simulink model "BiNode2016a"  (R2016a)
settings: Solver=ode4  StartTime=0.0  StopTime=6  FixedStep=tstep  RelTol=1e-3
PreLoadFcn:
  | xred=rednoise(20*1000)
model workspace (MAT data in the model file):
  P1 = Simulink.Parameter
  P1.Value = 4.5
  P1.DataType = 'auto'
  P1.Dimensions = [1 1]
  P2 = Simulink.Parameter
  P2.Value = 0
  P2.DataType = 'auto'
  P2.Dimensions = [1 1]
  V = Simulink.Parameter
  V.Value = 0.5
  V.DataType = 'auto'
  V.Dimensions = [1 1]
  e0 = Simulink.Parameter
  e0.Value = 2.5
  e0.DataType = 'auto'
  e0.Dimensions = [1 1]
  kp = Simulink.Parameter
  kp.Value = 0.1
  kp.DataType = 'auto'
  kp.Dimensions = [1 1]
  r = Simulink.Parameter
  r.Value = 1.12
  r.DataType = 'auto'
  r.Dimensions = [1 1]
  tao = Simulink.Parameter
  tao.Value = 0.01
  tao.DataType = 'auto'
  tao.Dimensions = [1 1]
  tstep = Simulink.Parameter
  tstep.Value = 0.0001
  tstep.DataType = 'auto'
  tstep.Dimensions = [1 1]
  v0 = Simulink.Parameter
  v0.Value = 5
  v0.DataType = 'auto'
  v0.Dimensions = [1 1]
libraries: commnoisgen2 x2
settings Model: Creator=u0085294  LastModifiedBy=mchehelc
settings DataIOCC: LimitDataPoints=on  SaveFormat=Array
settings OptimizationCC: ExpressionDepthLimit=2147483647
settings DebuggingCC: UnderspecifiedInitializationDetection=Classic  MergeDetectMultiDrivingBlocksExec=none  SolverPrmCheckMsg=warning  StateNameClashWarn=warning
settings HardwareCC: ProdBitPerPointer=32  ProdLargestAtomicFloat=None  ProdIntDivRoundTo=Undefined  ProdEndianess=Unspecified  ProdWordSize=32  ProdHWDeviceType=32-bit Generic
settings ModelReferenceCC: PropagateSignalLabelsOutOfModel=off
settings ConfigComp: CovModelRefEnable=Off

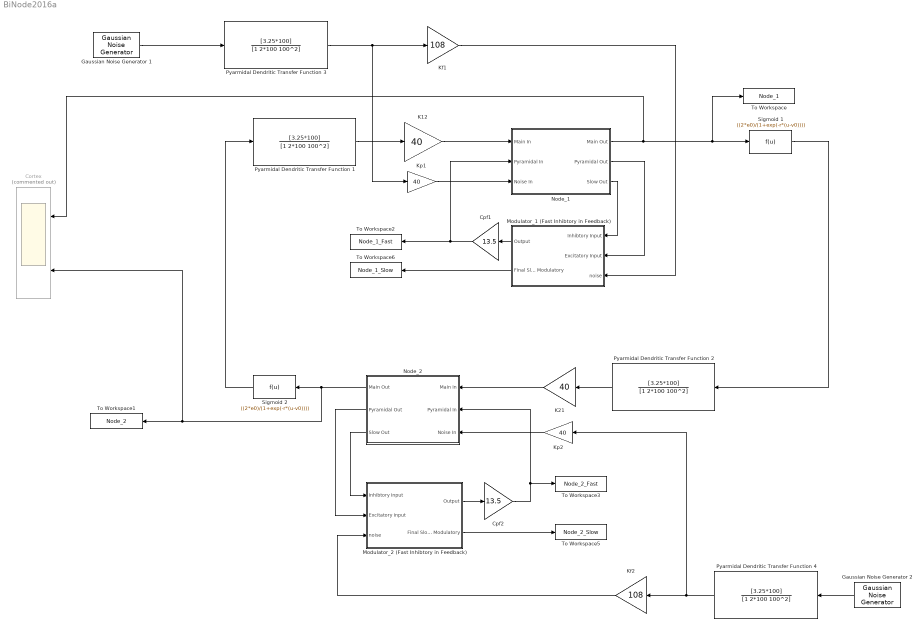
== system BiNode2016a ==
  Cortex : Scope  Commented=on  NumInputPorts=2
  Cpf1 : Gain  Gain=13.5
  Cpf2 : Gain  Gain=13.5
  Gaussian Noise Generator 1 : commnoisgen2/Gaussian Noise Generator  m=P1  d=V  s=44  Ts=tstep  frameBased=off  sampPerFrame=1  orient=off  outDataType=double
  Gaussian Noise Generator 2 : commnoisgen2/Gaussian Noise Generator  m=P2  d=V  s=41  Ts=tstep  frameBased=off  sampPerFrame=1  orient=off  outDataType=double
  K12 : Gain  Gain=40
  K21 : Gain  Gain=40
  Kf1 : Gain  Gain=108
  Kf2 : Gain  Gain=108
  Kp1 : Gain  Gain=40
  Kp2 : Gain  Gain=40
  Modulator_1 (Fast Inhibtory in Feedback) : Subsystem
  Modulator_2 (Fast Inhibtory in Feedback) : Subsystem
  Node_1 : Subsystem
  Node_2 : Subsystem
  Pyarmidal Dendritic Transfer Function 1 : TransferFcn  Numerator=[3.25*100]  Denominator=[1 2*100 100^2]
  Pyarmidal Dendritic Transfer Function 2 : TransferFcn  Numerator=[3.25*100]  Denominator=[1 2*100 100^2]
  Pyarmidal Dendritic Transfer Function 3 : TransferFcn  Numerator=[3.25*100]  Denominator=[1 2*100 100^2]
  "Pyarmidal Dendritic Transfer Function 4 " : TransferFcn  Numerator=[3.25*100]  Denominator=[1 2*100 100^2]
  Sigmoid 1 : Fcn  Expr=((2*e0)/(1+exp(-r*(u-v0))))
      mask Display: plot(1./(1+exp(-0.75.*([1:25]-12))))
  Sigmoid 2 : Fcn  Expr=((2*e0)/(1+exp(-r*(u-v0))))
      mask Display: plot(1./(1+exp(-0.75.*([1:25]-12))))
  To Workspace : ToWorkspace  VariableName=Node_1  SampleTime=-1
  To Workspace1 : ToWorkspace  VariableName=Node_2  SampleTime=-1
  To Workspace2 : ToWorkspace  VariableName=Node_1_Fast  SampleTime=-1
  To Workspace3 : ToWorkspace  VariableName=Node_2_Fast  SampleTime=-1
  To Workspace5 : ToWorkspace  VariableName=Node_2_Slow  SampleTime=-1
  To Workspace6 : ToWorkspace  VariableName=Node_1_Slow  SampleTime=-1
  wires:
  Node_1/1(Main Out) -> To Workspace/1, Sigmoid 1/1, Cortex/1
  Node_2/1(Main Out) -> Sigmoid 2/1, Cortex/2, To Workspace1/1
  Modulator_1 (Fast Inhibtory in Feedback)/1(Output) -> Cpf1/1
  Node_1/2(Pyramidal Out) -> Modulator_1 (Fast Inhibtory in Feedback)/2(Excitatory Input)
  Cpf1/1 -> Node_1/2(Pyramidal In), To Workspace2/1
  Modulator_2 (Fast Inhibtory in Feedback)/1(Output) -> Cpf2/1
  Node_2/2(Pyramidal Out) -> Modulator_2 (Fast Inhibtory in Feedback)/2(Excitatory Input)
  Sigmoid 1/1 -> Pyarmidal Dendritic Transfer Function 2/1
  Modulator_2 (Fast Inhibtory in Feedback)/2(Final Slow Modulatory) -> To Workspace5/1
  Modulator_1 (Fast Inhibtory in Feedback)/2(Final Slow Modulatory) -> To Workspace6/1
  Node_1/3(Slow Out) -> Modulator_1 (Fast Inhibtory in Feedback)/1(Inhibtory Input)
  Node_2/3(Slow Out) -> Modulator_2 (Fast Inhibtory in Feedback)/1(Inhibtory Input)
  Pyarmidal Dendritic Transfer Function 2/1 -> K21/1
  Kf2/1 -> Modulator_2 (Fast Inhibtory in Feedback)/3(noise)
  Gaussian Noise Generator 2/1 -> "Pyarmidal Dendritic Transfer Function 4 "/1
  "Pyarmidal Dendritic Transfer Function 4 "/1 -> Kp2/1, Kf2/1
  Pyarmidal Dendritic Transfer Function 1/1 -> K12/1
  Sigmoid 2/1 -> Pyarmidal Dendritic Transfer Function 1/1
  Gaussian Noise Generator 1/1 -> Pyarmidal Dendritic Transfer Function 3/1
  Pyarmidal Dendritic Transfer Function 3/1 -> Kf1/1, Kp1/1
  Kf1/1 -> Modulator_1 (Fast Inhibtory in Feedback)/3(noise)
  Cpf2/1 -> Node_2/2(Pyramidal In), To Workspace3/1
  K21/1 -> Node_2/1(Main In)
  Kp2/1 -> Node_2/3(Noise In)
  Kp1/1 -> Node_1/3(Noise In)
  K12/1 -> Node_1/1(Main In)

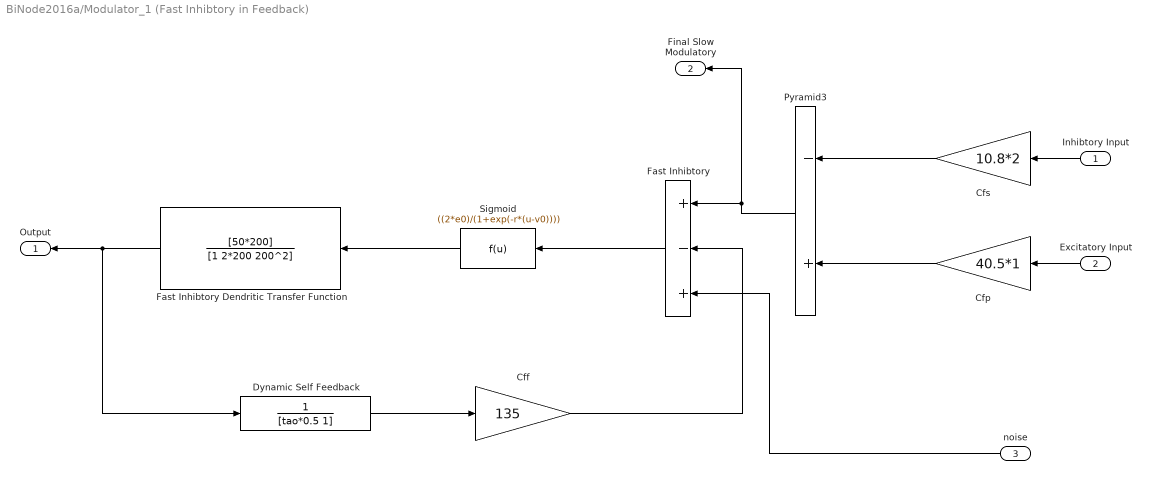
== system BiNode2016a/Modulator_1 (Fast Inhibtory in Feedback) ==
  Inhibtory Input : Inport
  Excitatory Input : Inport  Port=2
  noise : Inport  Port=3
  Cff : Gain  Gain=135
  Cfp : Gain  Gain=40.5*1
  Cfs : Gain  Gain=10.8*2
  Dynamic Self Feedback : TransferFcn  Numerator=1  Denominator=[tao*0.5 1]
  Fast Inhibtory : Sum  Inputs=+-+
  Fast Inhibtory Dendritic Transfer Function : TransferFcn  Numerator=[50*200]  Denominator=[1 2*200 200^2]
  Pyramid3 : Sum  Inputs=-+
  Sigmoid : Fcn  Expr=((2*e0)/(1+exp(-r*(u-v0))))
      mask Display: plot(1./(1+exp(-0.75.*([1:25]-12))))
  Output : Outport
  Final Slow Modulatory : Outport  Port=2
  wires:
  Inhibtory Input/1 -> Cfs/1
  Cff/1 -> Fast Inhibtory/2
  Cfp/1 -> Pyramid3/2
  Fast Inhibtory Dendritic Transfer Function/1 -> Dynamic Self Feedback/1, Output/1
  Dynamic Self Feedback/1 -> Cff/1
  noise/1 -> Fast Inhibtory/3
  Excitatory Input/1 -> Cfp/1
  Pyramid3/1 -> Fast Inhibtory/1, Final Slow Modulatory/1
  Fast Inhibtory/1 -> Sigmoid/1
  Cfs/1 -> Pyramid3/1
  Sigmoid/1 -> Fast Inhibtory Dendritic Transfer Function/1

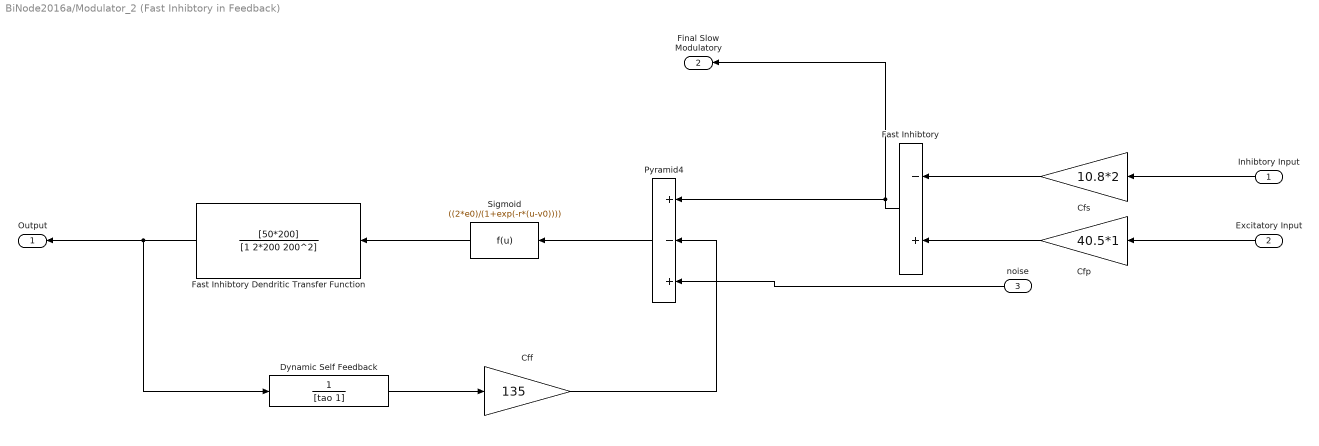
== system BiNode2016a/Modulator_2 (Fast Inhibtory in Feedback) ==
  Inhibtory Input : Inport
  Excitatory Input : Inport  Port=2
  noise : Inport  Port=3
  Cff : Gain  Gain=135
  Cfp : Gain  Gain=40.5*1
  Cfs : Gain  Gain=10.8*2
  Dynamic Self Feedback : TransferFcn  Numerator=1  Denominator=[tao 1]
  Fast Inhibtory : Sum  Inputs=-+
  Fast Inhibtory Dendritic Transfer Function : TransferFcn  Numerator=[50*200]  Denominator=[1 2*200 200^2]
  Pyramid4 : Sum  Inputs=+-+
  Sigmoid : Fcn  Expr=((2*e0)/(1+exp(-r*(u-v0))))
      mask Display: plot(1./(1+exp(-0.75.*([1:25]-12))))
  Output : Outport
  Final Slow Modulatory : Outport  Port=2
  wires:
  Inhibtory Input/1 -> Cfs/1
  Cff/1 -> Pyramid4/2
  Cfp/1 -> Fast Inhibtory/2
  Fast Inhibtory Dendritic Transfer Function/1 -> Dynamic Self Feedback/1, Output/1
  Dynamic Self Feedback/1 -> Cff/1
  Cfs/1 -> Fast Inhibtory/1
  Excitatory Input/1 -> Cfp/1
  Sigmoid/1 -> Fast Inhibtory Dendritic Transfer Function/1
  Pyramid4/1 -> Sigmoid/1
  Fast Inhibtory/1 -> Pyramid4/1, Final Slow Modulatory/1
  noise/1 -> Pyramid4/3

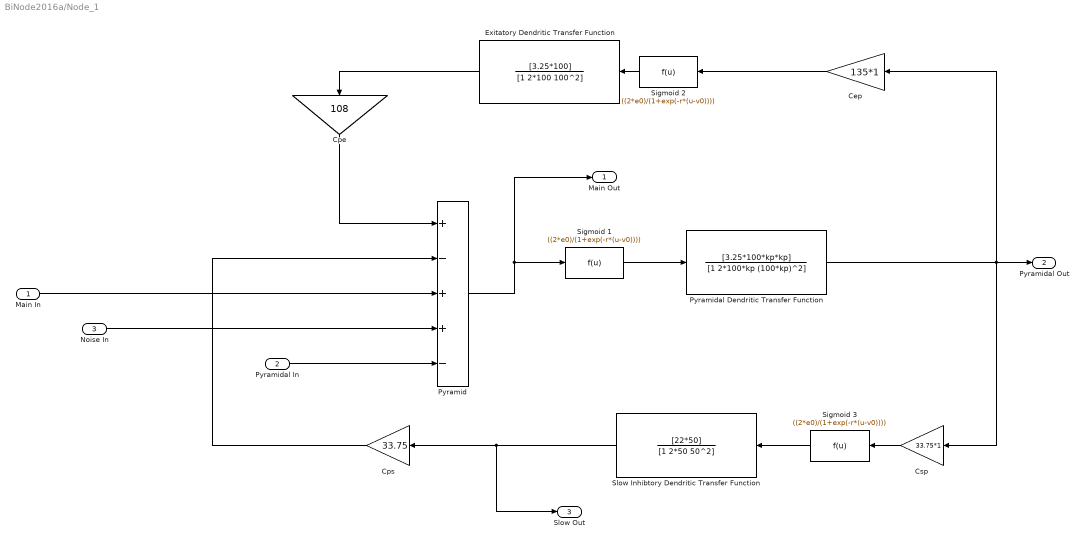
== system BiNode2016a/Node_1 ==
  Main In : Inport
  Pyramidal In : Inport  Port=2
  Noise In : Inport  Port=3
  Cep : Gain  Gain=135*1
  Cpe : Gain  Gain=108
  Cps : Gain  Gain=33.75
  Csp : Gain  Gain=33.75*1
  Exitatory Dendritic Transfer Function : TransferFcn  Numerator=[3.25*100]  Denominator=[1 2*100 100^2]
  Pyramid : Sum  Inputs=+-++-
  Pyramidal Dendritic Transfer Function : TransferFcn  Numerator=[3.25*100*kp*kp]  Denominator=[1 2*100*kp (100*kp)^2]
  Sigmoid 1 : Fcn  Expr=((2*e0)/(1+exp(-r*(u-v0))))
      mask Display: plot(1./(1+exp(-0.75.*([1:25]-12))))
  Sigmoid 2 : Fcn  Expr=((2*e0)/(1+exp(-r*(u-v0))))
      mask Display: plot(1./(1+exp(-0.75.*([1:25]-12))))
  Sigmoid 3 : Fcn  Expr=((2*e0)/(1+exp(-r*(u-v0))))
      mask Display: plot(1./(1+exp(-0.75.*([1:25]-12))))
  Slow Inhibtory Dendritic Transfer Function : TransferFcn  Numerator=[22*50]  Denominator=[1 2*50 50^2]
  Main Out : Outport
  Pyramidal Out : Outport  Port=2
  Slow Out : Outport  Port=3
  wires:
  Pyramidal Dendritic Transfer Function/1 -> Pyramidal Out/1, Cep/1, Csp/1
  Pyramid/1 -> Main Out/1, Sigmoid 1/1
  Sigmoid 1/1 -> Pyramidal Dendritic Transfer Function/1
  Exitatory Dendritic Transfer Function/1 -> Cpe/1
  Csp/1 -> Sigmoid 3/1
  Cps/1 -> Pyramid/2
  Cep/1 -> Sigmoid 2/1
  Slow Inhibtory Dendritic Transfer Function/1 -> Slow Out/1, Cps/1
  Sigmoid 2/1 -> Exitatory Dendritic Transfer Function/1
  Cpe/1 -> Pyramid/1
  Main In/1 -> Pyramid/3
  Sigmoid 3/1 -> Slow Inhibtory Dendritic Transfer Function/1
  Pyramidal In/1 -> Pyramid/5
  Noise In/1 -> Pyramid/4

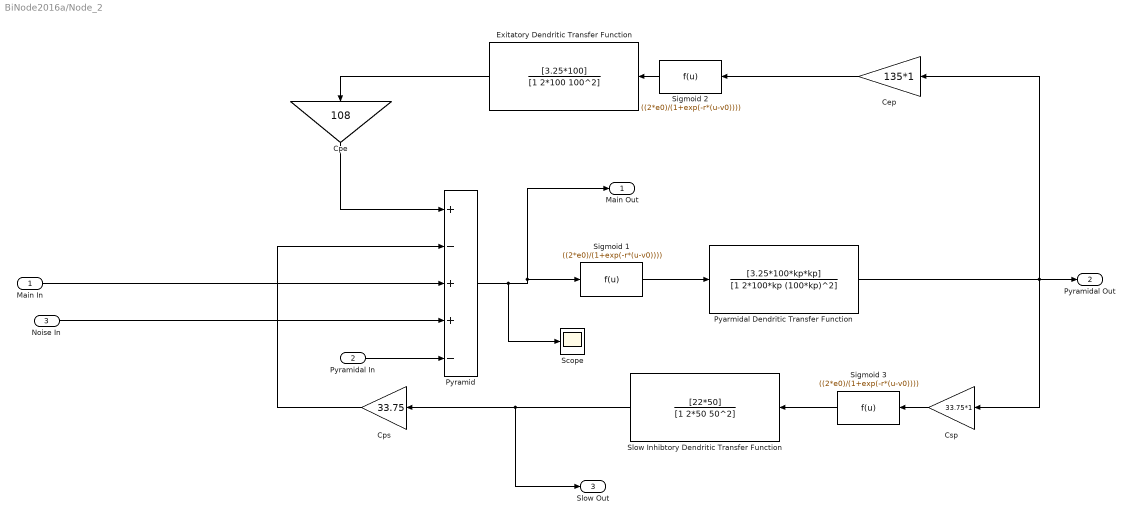
== system BiNode2016a/Node_2 ==
  Main In : Inport
  Pyramidal In : Inport  Port=2
  Noise In : Inport  Port=3
  Cep : Gain  Gain=135*1
  Cpe : Gain  Gain=108
  Cps : Gain  Gain=33.75
  Csp : Gain  Gain=33.75*1
  Exitatory Dendritic Transfer Function : TransferFcn  Numerator=[3.25*100]  Denominator=[1 2*100 100^2]
  Pyarmidal Dendritic Transfer Function : TransferFcn  Numerator=[3.25*100*kp*kp]  Denominator=[1 2*100*kp (100*kp)^2]
  Pyramid : Sum  Inputs=+-++-
  Scope : Scope
  Sigmoid 1 : Fcn  Expr=((2*e0)/(1+exp(-r*(u-v0))))
      mask Display: plot(1./(1+exp(-0.75.*([1:25]-12))))
  Sigmoid 2 : Fcn  Expr=((2*e0)/(1+exp(-r*(u-v0))))
      mask Display: plot(1./(1+exp(-0.75.*([1:25]-12))))
  Sigmoid 3 : Fcn  Expr=((2*e0)/(1+exp(-r*(u-v0))))
      mask Display: plot(1./(1+exp(-0.75.*([1:25]-12))))
  Slow Inhibtory Dendritic Transfer Function : TransferFcn  Numerator=[22*50]  Denominator=[1 2*50 50^2]
  Main Out : Outport
  Pyramidal Out : Outport  Port=2
  Slow Out : Outport  Port=3
  wires:
  Pyarmidal Dendritic Transfer Function/1 -> Pyramidal Out/1, Cep/1, Csp/1
  Pyramid/1 -> Scope/1, Main Out/1, Sigmoid 1/1
  Sigmoid 1/1 -> Pyarmidal Dendritic Transfer Function/1
  Exitatory Dendritic Transfer Function/1 -> Cpe/1
  Csp/1 -> Sigmoid 3/1
  Cps/1 -> Pyramid/2
  Cep/1 -> Sigmoid 2/1
  Sigmoid 3/1 -> Slow Inhibtory Dendritic Transfer Function/1
  Sigmoid 2/1 -> Exitatory Dendritic Transfer Function/1
  Cpe/1 -> Pyramid/1
  Main In/1 -> Pyramid/3
  Slow Inhibtory Dendritic Transfer Function/1 -> Slow Out/1, Cps/1
  Pyramidal In/1 -> Pyramid/5
  Noise In/1 -> Pyramid/4
